simulink model "gm_signalSim"  (R2023b)
settings: Solver=VariableStepAuto  StartTime=0.0  StopTime=0.1  RelTol=1e-3
undefined symbols (not defined in the file or in its folder): f, fs
libraries: hdlsllib x3, dspsrcs4 x2, dspfdesign x1
settings Model: Creator=31651  LastModifiedBy=31651
settings OptimizationCC: BlockReduction=off  ConditionallyExecuteInputs=off
settings DebuggingCC: InheritedTsInSrcMsg=none

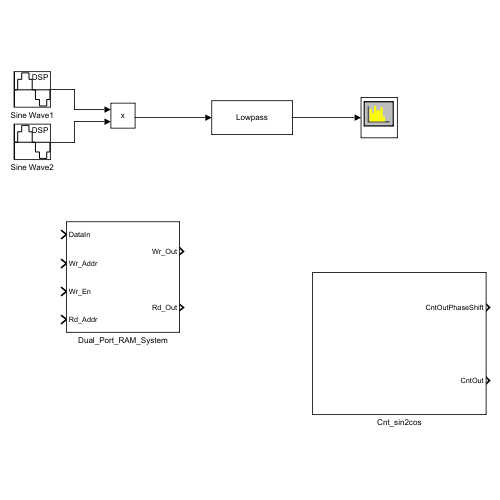
[thumbnail: Simulink's stored preview of the top-level diagram]
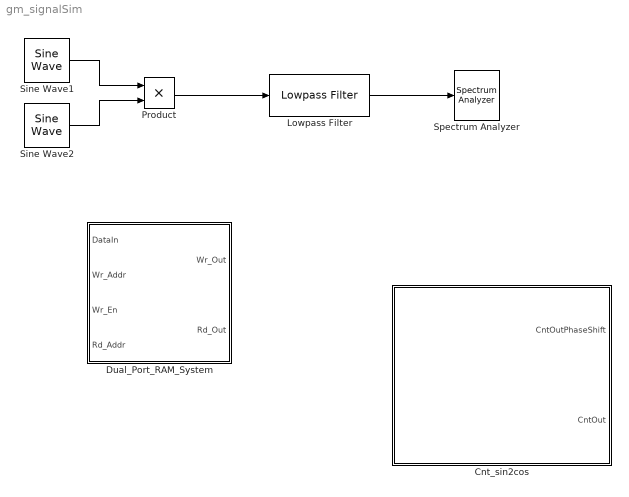
== system gm_signalSim ==
  Cnt_sin2cos : Subsystem
  Dual_Port_RAM_System : Subsystem
  Lowpass Filter : dspfdesign/Lowpass Filter  FilterType=FIR  DesignForMinimumOrder=on  FilterOrder=50  PassbandFrequency=1000  StopbandFrequency=1500  PassbandRipple=0.1  StopbandAttenuation=80  SampleRateMode=Specify on dialog  SampleRate=fs  SimulateUsing=Interpreted execution  roundingMode=Floor  coeffsDataTypeStr=fixdt(1,16)
  Product : Product
  Sine Wave1 : dspsrcs4/Sine Wave  Amplitude=2  Frequency=f  Phase=pi/2  SampleMode=Discrete  OutComplex=Real  CompMethod=Trigonometric fcn  TableSize=Speed  SampleTime=1/fs  SamplesPerFrame=1  ResetState=Restart at time zero  OutputFrames=off  dataType=double  wordLen=16  udDataType=sfix(16)  fracBitsMode=Best precision  numFracBits=15  OutDataTypeStr=double  LastOutDataTypeStr=double
  Sine Wave2 : dspsrcs4/Sine Wave  Amplitude=2  Frequency=f  Phase=-pi/6  SampleMode=Discrete  OutComplex=Real  CompMethod=Trigonometric fcn  TableSize=Speed  SampleTime=1/fs  SamplesPerFrame=1  ResetState=Restart at time zero  OutputFrames=off  dataType=double  wordLen=16  udDataType=sfix(16)  fracBitsMode=Best precision  numFracBits=15  OutDataTypeStr=double  LastOutDataTypeStr=double
  Spectrum Analyzer : SpectrumAnalyzer  WindowPosition=[560.000000,290.000000,800.000000,500.000000,]  Visible=on  ScopeFrameLocation=window  YLimits=[-186.93079374,54.1584696]
  wires:
  Lowpass Filter/1 -> Spectrum Analyzer/1
  Product/1 -> Lowpass Filter/1
  Sine Wave2/1 -> Product/2
  Sine Wave1/1 -> Product/1

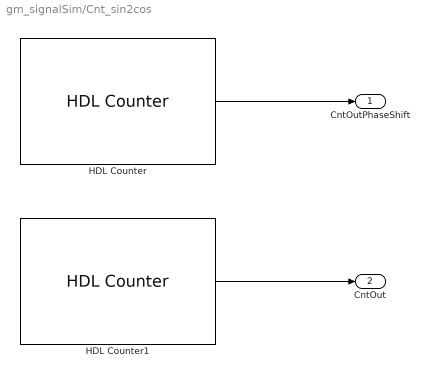
== system gm_signalSim/Cnt_sin2cos ==
  HDL Counter : hdlsllib/Sources/HDL Counter  CountType=Count limited  CountInit=325  CountStep=1  CountMax=3250  CountFromType=Specify  CountFrom=1  CountResetPort=off  CountLoadPort=off  CountEnbPort=off  CountDirPort=off  CountHitOutputPort=off  CountDataType=Unsigned  CountWordLen=16  CountFracLen=0  CountSampTime=1
  HDL Counter1 : hdlsllib/Sources/HDL Counter  CountType=Count limited  CountInit=1  CountStep=1  CountMax=3250  CountFromType=Specify  CountFrom=1  CountResetPort=off  CountLoadPort=off  CountEnbPort=off  CountDirPort=off  CountHitOutputPort=off  CountDataType=Unsigned  CountWordLen=16  CountFracLen=0  CountSampTime=1
  CntOutPhaseShift : Outport  VectorParamsAs1DForOutWhenUnconnected=off
  CntOut : Outport  Port=2  VectorParamsAs1DForOutWhenUnconnected=off
  wires:
  HDL Counter1/1 -> CntOut/1
  HDL Counter/1 -> CntOutPhaseShift/1

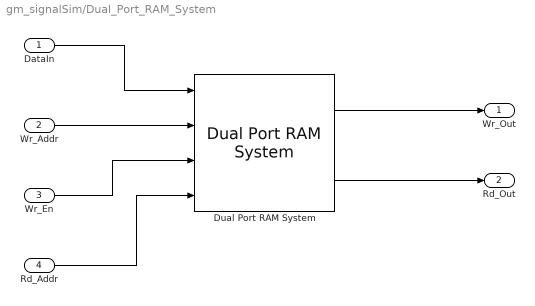
== system gm_signalSim/Dual_Port_RAM_System ==
  DataIn : Inport  OutDataTypeStr=uint16
  Wr_Addr : Inport  Port=2  OutDataTypeStr=uint16
  Wr_En : Inport  Port=3  OutDataTypeStr=boolean
  Rd_Addr : Inport  Port=4  OutDataTypeStr=uint16
  Dual Port RAM System : hdlsllib/HDL RAMs/Dual Port RAM System  RAMType=Dual port  AsyncRead=on  WriteOutputValue=New data  RAMInitialValue=0  allowBusInputs=off  WritesHaveOutput=on  NumReads=0  NumWrites=1  SimulateUsing=Code generation
  Wr_Out : Outport  OutDataTypeStr=uint16
  Rd_Out : Outport  Port=2  OutDataTypeStr=uint16
  wires:
  Rd_Addr/1 -> Dual Port RAM System/4
  DataIn/1 -> Dual Port RAM System/1
  Wr_Addr/1 -> Dual Port RAM System/2
  Dual Port RAM System/2 -> Rd_Out/1
  Dual Port RAM System/1 -> Wr_Out/1
  Wr_En/1 -> Dual Port RAM System/3
